simulink subsystem "PID_Mathmatical"  (R2023a)
settings: Solver=VariableStepAuto  StartTime=0.0  StopTime=10.0  RelTol=1e-3

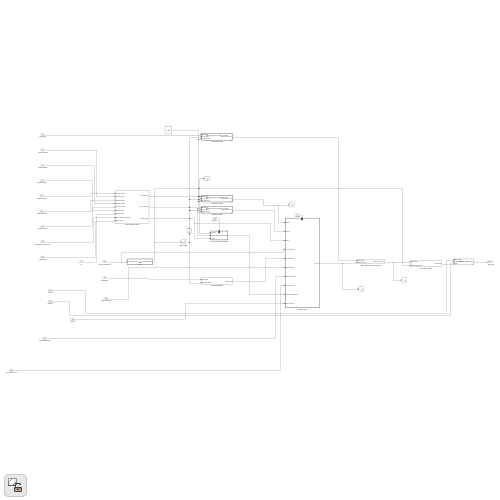
[thumbnail: Simulink's stored preview of the top-level diagram]
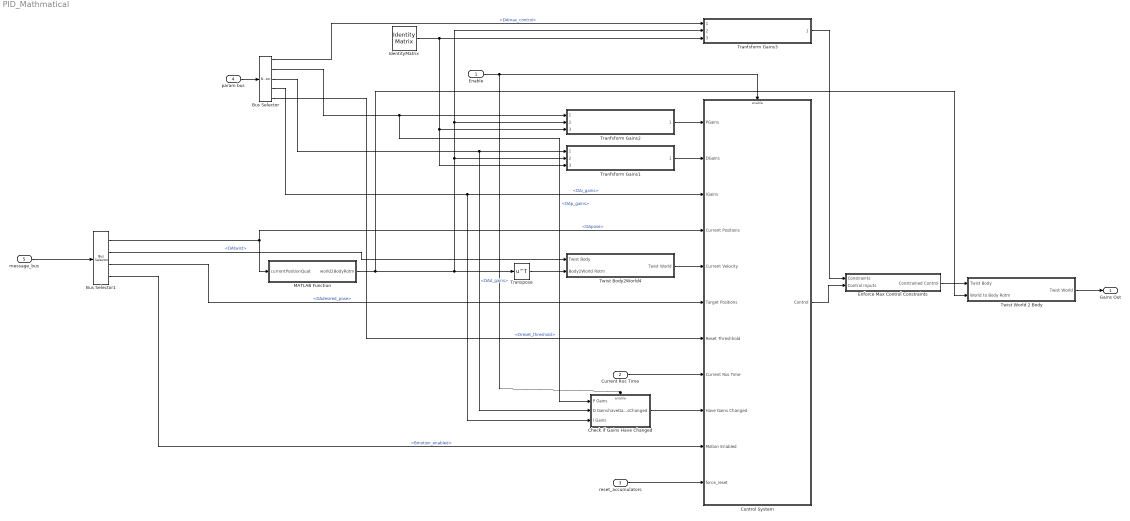
== system PID_Mathmatical ==
  Enable : Inport
  Current Ros Time : Inport  Port=2
  reset_accumulators : Inport  Port=3
  param bus : Inport  Port=4
  message_bus : Inport  Port=5
  Bus Selector : BusSelector  OutputSignals=DAmax_control,DAp_gains,DAd_gains,DAi_gains,Dreset_threshold
  Bus Selector1 : BusSelector  OutputSignals=current_state.DApose,current_state.DAtwist,desired_pose.DAdesired_pose,Bmotion_enabled
  Check if Gains Have Changed : Subsystem
  Control System : Subsystem
  Enforce Max Control Constraints : Subsystem
  IdentityMatrix : IdentityMatrix  OutputDimensions=3
  MATLAB Function : MATLAB Function  TreatAsAtomicUnit=on
  Tranfsform Gains1 : Subsystem  TreatAsAtomicUnit=on  ReferencedSubsystem=Tranfsform_Linear_Gains_To_World
  Tranfsform Gains2 : Subsystem  TreatAsAtomicUnit=on  ReferencedSubsystem=Tranfsform_Linear_Gains_To_World
  Tranfsform Gains3 : Subsystem  TreatAsAtomicUnit=on  ReferencedSubsystem=Tranfsform_Linear_Gains_To_World
  Transpose : Math  Operator=transpose
  Twist Body2World4 : Subsystem
  Twist World 2 Body : Subsystem
  Gains Out : Outport
  wires:
  Check if Gains Have Changed/1(haveGainsChanged) -> Control System/9(Have Gains Changed)
  Enable/1 -> Check if Gains Have Changed/Enable, Control System/Enable
  Bus Selector1/3 -> Control System/6(Target Positions)  "<DAdesired_pose>"
  Current Ros Time/1 -> Control System/8(Current Ros Time)
  Enforce Max Control Constraints/1(Constrained Control) -> Twist World 2 Body/1(Twist Body)
  Control System/1(Control) -> Enforce Max Control Constraints/2(Control Inputs)
  IdentityMatrix/1 -> Tranfsform Gains3/3, Tranfsform Gains2/3, Tranfsform Gains1/3
  Twist Body2World4/1(Twist World) -> Control System/5(Current Velocity)
  Tranfsform Gains1/1 -> Control System/2(DGains)
  Tranfsform Gains3/1 -> Enforce Max Control Constraints/1(Constraints)
  Tranfsform Gains2/1 -> Control System/1(PGains)
  Twist World 2 Body/1(Twist World) -> Gains Out/1
  MATLAB Function/1(world2BodyRotm) -> Transpose/1, Tranfsform Gains1/2, Tranfsform Gains2/2, Tranfsform Gains3/2, Twist World 2 Body/2(World to Body Rotm)
  Bus Selector/4 -> Control System/3(IGains), Check if Gains Have Changed/3(I Gains)  "<DAi_gains>"
  Transpose/1 -> Twist Body2World4/2(Body2World Rotm)
  reset_accumulators/1 -> Control System/11(force_reset)
  param bus/1 -> Bus Selector/1
  Bus Selector/1 -> Tranfsform Gains3/1  "<DAmax_control>"
  Bus Selector/2 -> Tranfsform Gains2/1, Check if Gains Have Changed/1(P Gains)  "<DAp_gains>"
  Bus Selector/3 -> Tranfsform Gains1/1, Check if Gains Have Changed/2(D Gains)  "<DAd_gains>"
  Bus Selector/5 -> Control System/7(Reset Threshhold)  "<Dreset_threshold>"
  message_bus/1 -> Bus Selector1/1
  Bus Selector1/1 -> Control System/4(Current Positions), MATLAB Function/1(currentPositionQuat)  "<DApose>"
  Bus Selector1/2 -> Twist Body2World4/1(Twist Body)  "<DAtwist>"
  Bus Selector1/4 -> Control System/10(Motion Enabled)  "<Bmotion_enabled>"

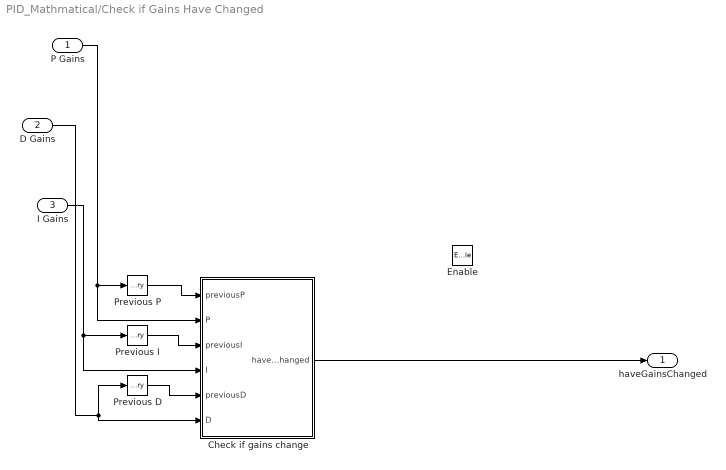
== system PID_Mathmatical/Check if Gains Have Changed ==
  P Gains : Inport
  D Gains : Inport  Port=2
  I Gains : Inport  Port=3
  Enable : EnablePort
  Check if gains change : MATLAB Function  TreatAsAtomicUnit=on
  Previous D : Memory  InheritSampleTime=on
  Previous I : Memory  InheritSampleTime=on
  Previous P : Memory  InheritSampleTime=on
  haveGainsChanged : Outport
  wires:
  Check if gains change/1(haveGainsChanged) -> haveGainsChanged/1
  D Gains/1 -> Check if gains change/6(D), Previous D/1
  Previous D/1 -> Check if gains change/5(previousD)
  P Gains/1 -> Previous P/1, Check if gains change/2(P)
  Previous P/1 -> Check if gains change/1(previousP)
  Previous I/1 -> Check if gains change/3(previousI)
  I Gains/1 -> Previous I/1, Check if gains change/4(I)

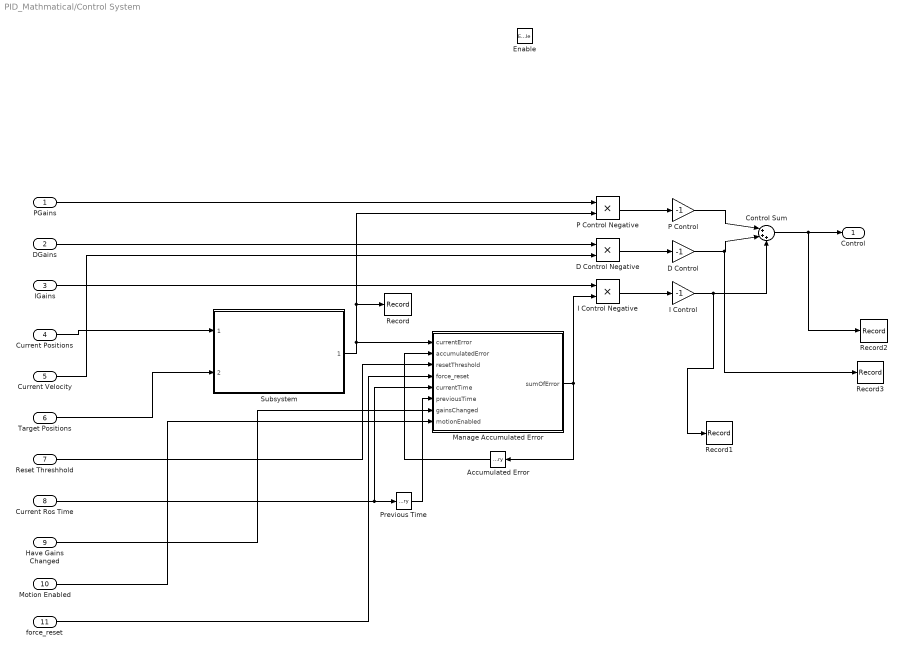
== system PID_Mathmatical/Control System ==
  PGains : Inport
  DGains : Inport  Port=2
  IGains : Inport  Port=3
  Current Positions : Inport  Port=4
  Current Velocity : Inport  Port=5
  Target Positions : Inport  Port=6
  Reset Threshhold : Inport  Port=7
  Current Ros Time : Inport  Port=8
  Have Gains Changed : Inport  Port=9
  Motion Enabled : Inport  Port=10
  force_reset : Inport  Port=11
  Enable : EnablePort
  Accumulated Error : Memory  InheritSampleTime=on
  Control Sum : Sum  Inputs=|+++
  D Control : Gain  Gain=-1
  D Control Negative : Product
  I Control : Gain  Gain=-1
  I Control Negative : Product
  Manage Accumulated Error : MATLAB Function  TreatAsAtomicUnit=on
  P Control : Gain  Gain=-1
  P Control Negative : Product
  Previous Time : Memory  InitialCondition=-1  InheritSampleTime=on
  Record : Record  FileSettingsInternal="{\"entries\":[{\"content\":{\"excelSettings\":{\"content\":{},\"type\":\"Streamout.ExcelSettings\"}},\"type\":\"Streamout.FileSettingStorage\",\"uuid\":\"\"}],\"packageUris\":[\"http:\\/\\/schema.mathworks.com\\/mf0\\/streamout_blocks\\/R2020a\"],\"version\":\"1.0\"}"  Layout=[1 1]  SignalsInternal="{\"entries\":[{\"content\":{\"signals\":[{\"content\":{\"blockPath\":[],\"dimensions\":[1,6],\"domain\":\"\",\"hasChildren\":true,\"lineColor\":\"#22b573\",\"port\":1,\"signalID\":4990,\"signalName\":\"Normalize Error\"},\"type\":\"RecordBlkView.Signal\",\"uuid\":\"\"},{\"content\":{\"blockPath\":[],\"channel\":[1,1],\"dimensions\":[1,6],\"domain\":\"\",\"lineColor\":\"#0072bd\",\"parentID\":4990,\"port\":1,\"signalID\":4991,\"signalName\":\"Normalize Error\"} ...(+1249 chars)"  VisualizationBindings="{\"sparklinesplugin\":{\"info\":[{\"bindingParametersList\":[],\"subplotID\":1}]}}"
  Record1 : Record  FileSettingsInternal="{\"entries\":[{\"content\":{\"excelSettings\":{\"content\":{},\"type\":\"Streamout.ExcelSettings\"}},\"type\":\"Streamout.FileSettingStorage\",\"uuid\":\"\"}],\"packageUris\":[\"http:\\/\\/schema.mathworks.com\\/mf0\\/streamout_blocks\\/R2020a\"],\"version\":\"1.0\"}"  Layout=[1 1]  SignalsInternal="{\"entries\":[{\"content\":{\"signals\":[{\"content\":{\"blockPath\":[],\"dimensions\":[1,6],\"domain\":\"\",\"hasChildren\":true,\"lineColor\":\"#4dbeee\",\"port\":1,\"signalID\":5007,\"signalName\":\"I Control\"},\"type\":\"RecordBlkView.Signal\",\"uuid\":\"\"},{\"content\":{\"blockPath\":[],\"channel\":[1,1],\"dimensions\":[1,6],\"domain\":\"\",\"lineColor\":\"#b746ff\",\"parentID\":5007,\"port\":1,\"signalID\":5008,\"signalName\":\"I Control\"},\"type\":\"Rec ...(+1231 chars)"  VisualizationBindings="{\"sparklinesplugin\":{\"info\":[{\"bindingParametersList\":[],\"subplotID\":1}]}}"
  Record2 : Record  FileSettingsInternal="{\"entries\":[{\"content\":{\"excelSettings\":{\"content\":{},\"type\":\"Streamout.ExcelSettings\"}},\"type\":\"Streamout.FileSettingStorage\",\"uuid\":\"\"}],\"packageUris\":[\"http:\\/\\/schema.mathworks.com\\/mf0\\/streamout_blocks\\/R2020a\"],\"version\":\"1.0\"}"  Layout=[1 1]  SignalsInternal="{\"entries\":[{\"content\":{\"signals\":[{\"content\":{\"blockPath\":[],\"dimensions\":[1,6],\"domain\":\"\",\"hasChildren\":true,\"lineColor\":\"#7e2f8e\",\"port\":1,\"signalID\":5024,\"signalName\":\"Control Sum\"},\"type\":\"RecordBlkView.Signal\",\"uuid\":\"\"},{\"content\":{\"blockPath\":[],\"channel\":[1,1],\"dimensions\":[1,6],\"domain\":\"\",\"lineColor\":\"#b746ff\",\"parentID\":5024,\"port\":1,\"signalID\":5025,\"signalName\":\"Control Sum\"},\"type\": ...(+1221 chars)"  VisualizationBindings="{\"sparklinesplugin\":{\"info\":[{\"bindingParametersList\":[],\"subplotID\":1}]}}"
  Record3 : Record  FileSettingsInternal="{\"entries\":[{\"content\":{\"excelSettings\":{\"content\":{},\"type\":\"Streamout.ExcelSettings\"}},\"type\":\"Streamout.FileSettingStorage\",\"uuid\":\"\"}],\"packageUris\":[\"http:\\/\\/schema.mathworks.com\\/mf0\\/streamout_blocks\\/R2020a\"],\"version\":\"1.0\"}"  Layout=[1 1]  SignalsInternal="{\"entries\":[{\"content\":{\"signals\":[{\"content\":{\"blockPath\":[],\"dimensions\":[6],\"domain\":\"\",\"hasChildren\":true,\"lineColor\":\"#4dbeee\",\"port\":1,\"signalID\":5041,\"signalName\":\"D Control\"},\"type\":\"RecordBlkView.Signal\",\"uuid\":\"\"},{\"content\":{\"blockPath\":[],\"channel\":[1],\"dimensions\":[6],\"domain\":\"\",\"lineColor\":\"#a2142f\",\"parentID\":5041,\"port\":1,\"signalID\":5042,\"signalName\":\"D Control\"},\"type\":\"RecordBlk ...(+1181 chars)"  VisualizationBindings="{\"sparklinesplugin\":{\"info\":[{\"bindingParametersList\":[],\"subplotID\":1}]}}"
  Subsystem : Subsystem  ReferencedSubsystem=Normalize_Pose_Error
  Control : Outport
  wires:
  Target Positions/1 -> Subsystem/2
  Current Positions/1 -> Subsystem/1
  Subsystem/1 -> Manage Accumulated Error/1(currentError), P Control Negative/2, Record/1
  force_reset/1 -> Manage Accumulated Error/4(force_reset)
  Motion Enabled/1 -> Manage Accumulated Error/8(motionEnabled)
  Have Gains Changed/1 -> Manage Accumulated Error/7(gainsChanged)
  DGains/1 -> D Control Negative/1
  PGains/1 -> P Control Negative/1
  IGains/1 -> I Control Negative/1
  Current Ros Time/1 -> Manage Accumulated Error/5(currentTime), Previous Time/1
  Previous Time/1 -> Manage Accumulated Error/6(previousTime)
  Control Sum/1 -> Control/1, Record2/1
  I Control Negative/1 -> I Control/1
  Manage Accumulated Error/1(sumOfError) -> Accumulated Error/1, I Control Negative/2
  D Control/1 -> Control Sum/2, Record3/1
  Accumulated Error/1 -> Manage Accumulated Error/2(accumulatedError)
  P Control Negative/1 -> P Control/1
  D Control Negative/1 -> D Control/1
  P Control/1 -> Control Sum/1
  Current Velocity/1 -> D Control Negative/2
  I Control/1 -> Control Sum/3, Record1/1
  Reset Threshhold/1 -> Manage Accumulated Error/3(resetThreshold)

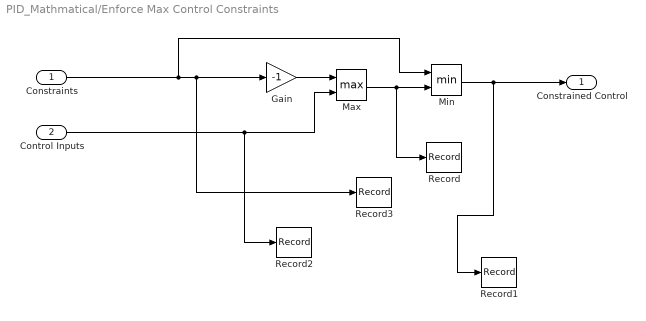
== system PID_Mathmatical/Enforce Max Control Constraints ==
  Constraints : Inport
  Control Inputs : Inport  Port=2
  Gain : Gain  Gain=-1
  Max : MinMax  Function=max  Inputs=2
  Min : MinMax  Inputs=2
  Record : Record  FileSettingsInternal="{\"entries\":[{\"content\":{\"excelSettings\":{\"content\":{},\"type\":\"Streamout.ExcelSettings\"}},\"type\":\"Streamout.FileSettingStorage\",\"uuid\":\"\"}],\"packageUris\":[\"http:\\/\\/schema.mathworks.com\\/mf0\\/streamout_blocks\\/R2020a\"],\"version\":\"1.0\"}"  Layout=[1 1]  SignalsInternal="{\"entries\":[{\"content\":{\"signals\":[{\"content\":{\"blockPath\":[],\"dimensions\":[1,6],\"domain\":\"\",\"hasChildren\":true,\"lineColor\":\"#b746ff\",\"port\":1,\"signalID\":5058,\"signalName\":\"Max\"},\"type\":\"RecordBlkView.Signal\",\"uuid\":\"\"},{\"content\":{\"blockPath\":[],\"channel\":[1,1],\"dimensions\":[1,6],\"domain\":\"\",\"lineColor\":\"#0072bd\",\"parentID\":5058,\"port\":1,\"signalID\":5059,\"signalName\":\"Max\"},\"type\":\"RecordBlkView.S ...(+1177 chars)"  VisualizationBindings="{\"sparklinesplugin\":{\"info\":[{\"bindingParametersList\":[],\"subplotID\":1}]}}"
  Record1 : Record  FileSettingsInternal="{\"entries\":[{\"content\":{\"excelSettings\":{\"content\":{},\"type\":\"Streamout.ExcelSettings\"}},\"type\":\"Streamout.FileSettingStorage\",\"uuid\":\"\"}],\"packageUris\":[\"http:\\/\\/schema.mathworks.com\\/mf0\\/streamout_blocks\\/R2020a\"],\"version\":\"1.0\"}"  Layout=[1 1]  SignalsInternal="{\"entries\":[{\"content\":{\"signals\":[{\"content\":{\"blockPath\":[],\"dimensions\":[1,6],\"domain\":\"\",\"hasChildren\":true,\"lineColor\":\"#ff13a6\",\"port\":1,\"signalID\":5075,\"signalName\":\"Min\"},\"type\":\"RecordBlkView.Signal\",\"uuid\":\"\"},{\"content\":{\"blockPath\":[],\"channel\":[1,1],\"dimensions\":[1,6],\"domain\":\"\",\"lineColor\":\"#0072bd\",\"parentID\":5075,\"port\":1,\"signalID\":5076,\"signalName\":\"Min\"},\"type\":\"RecordBlkView.S ...(+163 chars)"  VisualizationBindings="{\"sparklinesplugin\":{\"info\":[{\"bindingParametersList\":[],\"subplotID\":1}]}}"
  Record2 : Record  FileSettingsInternal="{\"entries\":[{\"content\":{\"excelSettings\":{\"content\":{},\"type\":\"Streamout.ExcelSettings\"}},\"type\":\"Streamout.FileSettingStorage\",\"uuid\":\"\"}],\"packageUris\":[\"http:\\/\\/schema.mathworks.com\\/mf0\\/streamout_blocks\\/R2020a\"],\"version\":\"1.0\"}"  Layout=[1 1]  SignalsInternal="{\"entries\":[{\"content\":{\"signals\":[{\"content\":{\"blockPath\":[],\"dimensions\":[1,6],\"domain\":\"\",\"hasChildren\":true,\"lineColor\":\"#22b573\",\"port\":1,\"signalID\":5087,\"signalName\":\"Control Inputs\"},\"type\":\"RecordBlkView.Signal\",\"uuid\":\"\"},{\"content\":{\"blockPath\":[],\"channel\":[1,1],\"dimensions\":[1,6],\"domain\":\"\",\"lineColor\":\"#77ac30\",\"parentID\":5087,\"port\":1,\"signalID\":5088,\"signalName\":\"Control Inputs\"},\" ...(+1254 chars)"  VisualizationBindings="{\"sparklinesplugin\":{\"info\":[{\"bindingParametersList\":[],\"subplotID\":1}]}}"
  Record3 : Record  FileSettingsInternal="{\"entries\":[{\"content\":{\"excelSettings\":{\"content\":{},\"type\":\"Streamout.ExcelSettings\"}},\"type\":\"Streamout.FileSettingStorage\",\"uuid\":\"\"}],\"packageUris\":[\"http:\\/\\/schema.mathworks.com\\/mf0\\/streamout_blocks\\/R2020a\"],\"version\":\"1.0\"}"  Layout=[1 1]  SignalsInternal="{\"entries\":[{\"content\":{\"signals\":[{\"content\":{\"blockPath\":[],\"dimensions\":[6],\"domain\":\"\",\"hasChildren\":true,\"lineColor\":\"#d95319\",\"port\":1,\"signalID\":5104,\"signalName\":\"Constraints\"},\"type\":\"RecordBlkView.Signal\",\"uuid\":\"\"},{\"content\":{\"blockPath\":[],\"channel\":[1],\"dimensions\":[6],\"domain\":\"\",\"lineColor\":\"#a2142f\",\"parentID\":5104,\"port\":1,\"signalID\":5105,\"signalName\":\"Constraints\"},\"type\":\"Recor ...(+1219 chars)"  VisualizationBindings="{\"sparklinesplugin\":{\"info\":[{\"bindingParametersList\":[],\"subplotID\":1}]}}"
  Constrained Control : Outport
  wires:
  Constraints/1 -> Gain/1, Record3/1, Min/1
  Max/1 -> Min/2, Record/1
  Control Inputs/1 -> Max/2, Record2/1
  Min/1 -> Constrained Control/1, Record1/1
  Gain/1 -> Max/1

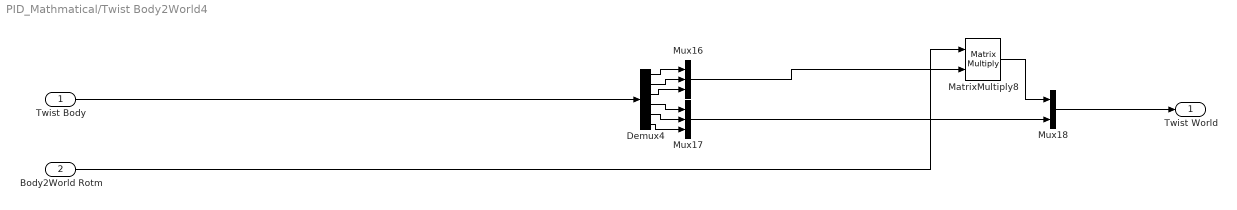
== system PID_Mathmatical/Twist Body2World4 ==
  Twist Body : Inport
  Body2World Rotm : Inport  Port=2
  Demux4 : Demux  Outputs=6
  MatrixMultiply8 : Product  Multiplication=Matrix(*)
  Mux16 : Mux  Inputs=3
  Mux17 : Mux  Inputs=3
  Mux18 : Mux  Inputs=2
  Twist World : Outport
  wires:
  Mux18/1 -> Twist World/1
  MatrixMultiply8/1 -> Mux18/1
  Body2World Rotm/1 -> MatrixMultiply8/1
  Demux4/3 -> Mux16/3
  Twist Body/1 -> Demux4/1
  Mux17/1 -> Mux18/2
  Demux4/5 -> Mux17/2
  Demux4/1 -> Mux16/1
  Demux4/6 -> Mux17/3
  Mux16/1 -> MatrixMultiply8/2
  Demux4/4 -> Mux17/1
  Demux4/2 -> Mux16/2

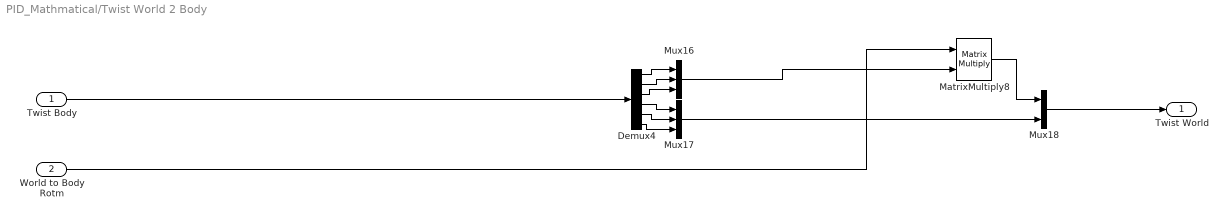
== system PID_Mathmatical/Twist World 2 Body ==
  Twist Body : Inport
  World to Body Rotm : Inport  Port=2
  Demux4 : Demux  Outputs=6
  MatrixMultiply8 : Product  Multiplication=Matrix(*)
  Mux16 : Mux  Inputs=3
  Mux17 : Mux  Inputs=3
  Mux18 : Mux  Inputs=2
  Twist World : Outport
  wires:
  World to Body Rotm/1 -> MatrixMultiply8/1
  Mux18/1 -> Twist World/1
  MatrixMultiply8/1 -> Mux18/1
  Demux4/3 -> Mux16/3
  Twist Body/1 -> Demux4/1
  Mux17/1 -> Mux18/2
  Demux4/5 -> Mux17/2
  Demux4/1 -> Mux16/1
  Demux4/6 -> Mux17/3
  Mux16/1 -> MatrixMultiply8/2
  Demux4/4 -> Mux17/1
  Demux4/2 -> Mux16/2

== matlab function PID_Mathmatical/Control System/Manage Accumulated Error ==
function sumOfError = fcn(currentError, accumulatedError, resetThreshold, force_reset, currentTime, previousTime, gainsChanged, motionEnabled)

deltaTime = 0;
if(previousTime <= 0)
    sumOfError = zeros(1,6);
    return 
else
    deltaTime = currentTime - previousTime;
end

sum = zeros(1,6);

%if gains get reset, reset accumulator
if(gainsChanged || ~motionEnabled)
   sumOfError = zeros(1,6);

   disp(gainsChanged)

   return
end

%check each degree of freedom
for i = 1:6
    sum(i) = (currentError(i)) * deltaTime + accumulatedError(i);

    if(abs(currentError(i)) > resetThreshold || force_reset)
        sum(i) = 0;
    end

    %reset if nan
    if(isnan(currentError(i)))
        sum(i) = 0;
    end

end

sumOfError = sum;

== matlab function PID_Mathmatical/MATLAB Function ==
function world2BodyRotm = fcn(currentPositionQuat)


world2BodyRotm = quat2rotm([currentPositionQuat(7), currentPositionQuat(4), currentPositionQuat(5), currentPositionQuat(6)]);

%fuk u matlab
world2BodyRotm = transpose(world2BodyRotm);

== matlab function PID_Mathmatical/Check if Gains Have Changed/Check if gains change ==
function haveGainsChanged  = fcn(previousP, P, previousI, I, previousD, D)


%check if P gains have changed
if(~isequal(P, previousP))
    haveGainsChanged = true;
    return
end


%check if  I gains have changed
if(~isequal(I, previousI))
    haveGainsChanged = true;
    return
end


%check if  D gains have changed
if(~isequal(D, previousD))
    haveGainsChanged = true;
    return
end

haveGainsChanged = false;
